simulink model "Quadcopter_State_model_Arduino"  (R2023b)
settings: Solver=VariableStepAuto  StartTime=0.0  StopTime=inf  FixedStep=0.00001  MinStep=0.001  RelTol=1e-3
model workspace (MAT data in the model file):
  DesiredPitchRoll : sugfis (value not decoded)
  DesiredThrust = sugfis
  DesiredThrust.Name = "fis"
  DesiredThrust.Type = "sugeno"
  DesiredThrust.AndMethod = "min"
  DesiredThrust.OrMethod = "max"
  DesiredThrust.FuzzyInferenceSystem.LocalImplicationMethod = "prod"
  DesiredThrust.FuzzyInferenceSystem.LocalAggregationMethod = "sum"
  DesiredThrust.FuzzyInferenceSystem.LocalDefuzzificationMethod = "wtaver"
  DesiredThrust.Inputs = fisvar
  DesiredThrust.Inputs.LocalName = "e_zdot"
  DesiredThrust.Inputs.Range = [-0.3 0.3]
  DesiredThrust.Inputs.EvalfisData.name = ' '
  DesiredThrust.Inputs.EvalfisData.range = [-0.3 0.3]
  DesiredThrust.Inputs.EvalfisData.mf(1).name = ' '
  DesiredThrust.Inputs.EvalfisData.mf(1).type = 'trimf'
  DesiredThrust.Inputs.EvalfisData.mf(1).params = [-0.45 -0.3 -0.15]
  DesiredThrust.Inputs.EvalfisData.mf(2).name = ' '
  DesiredThrust.Inputs.EvalfisData.mf(2).type = 'trimf'
  DesiredThrust.Inputs.EvalfisData.mf(2).params = [-0.3 -0.15 0]
  DesiredThrust.Inputs.EvalfisData.mf(3).name = ' '
  DesiredThrust.Inputs.EvalfisData.mf(3).type = 'trimf'
  DesiredThrust.Inputs.EvalfisData.mf(3).params = [-0.15 0 0.15]
  DesiredThrust.Inputs.EvalfisData.mf(4).name = ' '
  DesiredThrust.Inputs.EvalfisData.mf(4).type = 'trimf'
  DesiredThrust.Inputs.EvalfisData.mf(4).params = [0 0.15 0.3]
  DesiredThrust.Inputs.EvalfisData.mf(5).name = ' '
  DesiredThrust.Inputs.EvalfisData.mf(5).type = 'trimf'
  DesiredThrust.Inputs.EvalfisData.mf(5).params = [0.15 0.3 0.45]
  DesiredThrust.Inputs.LocalMembershipFunctions(1) = fismf
  DesiredThrust.Inputs.LocalMembershipFunctions(1).Function : function handle (value not decoded)
  DesiredThrust.Inputs.LocalMembershipFunctions(1).Parameters = [-0.45 -0.3 -0.15]
  DesiredThrust.Inputs.LocalMembershipFunctions(1).ParameterValueValidator : function handle (value not decoded)
  DesiredThrust.Inputs.LocalMembershipFunctions(1).NumParameters = 3
  DesiredThrust.Inputs.LocalMembershipFunctions(1).TypeStr = "trimf"
  DesiredThrust.Inputs.LocalMembershipFunctions(1).EvalfisData.name = ' '
  DesiredThrust.Inputs.LocalMembershipFunctions(1).EvalfisData.type = 'trimf'
  DesiredThrust.Inputs.LocalMembershipFunctions(1).EvalfisData.params = [-0.45 -0.3 -0.15]
  DesiredThrust.Inputs.LocalMembershipFunctions(1).fuzzy.internal.fis.MembershipFunction.LocalName = "StrongThrustDown"
  DesiredThrust.Inputs.LocalMembershipFunctions(1).UnmatchedInputArguments = struct()
  DesiredThrust.Inputs.LocalMembershipFunctions(2) = fismf
  DesiredThrust.Inputs.LocalMembershipFunctions(2).Function : function handle (value not decoded)
  DesiredThrust.Inputs.LocalMembershipFunctions(2).Parameters = [-0.3 -0.15 0]
  DesiredThrust.Inputs.LocalMembershipFunctions(2).ParameterValueValidator : function handle (value not decoded)
  DesiredThrust.Inputs.LocalMembershipFunctions(2).NumParameters = 3
  DesiredThrust.Inputs.LocalMembershipFunctions(2).TypeStr = "trimf"
  DesiredThrust.Inputs.LocalMembershipFunctions(2).EvalfisData.name = ' '
  DesiredThrust.Inputs.LocalMembershipFunctions(2).EvalfisData.type = 'trimf'
  DesiredThrust.Inputs.LocalMembershipFunctions(2).EvalfisData.params = [-0.3 -0.15 0]
  DesiredThrust.Inputs.LocalMembershipFunctions(2).fuzzy.internal.fis.MembershipFunction.LocalName = "MediumThrustDown"
  DesiredThrust.Inputs.LocalMembershipFunctions(2).UnmatchedInputArguments = struct()
  DesiredThrust.Inputs.LocalMembershipFunctions(3) = fismf
  DesiredThrust.Inputs.LocalMembershipFunctions(3).Function : function handle (value not decoded)
  DesiredThrust.Inputs.LocalMembershipFunctions(3).Parameters = [-0.15 0 0.15]
  DesiredThrust.Inputs.LocalMembershipFunctions(3).ParameterValueValidator : function handle (value not decoded)
  DesiredThrust.Inputs.LocalMembershipFunctions(3).NumParameters = 3
  DesiredThrust.Inputs.LocalMembershipFunctions(3).TypeStr = "trimf"
  DesiredThrust.Inputs.LocalMembershipFunctions(3).EvalfisData.name = ' '
  DesiredThrust.Inputs.LocalMembershipFunctions(3).EvalfisData.type = 'trimf'
  DesiredThrust.Inputs.LocalMembershipFunctions(3).EvalfisData.params = [-0.15 0 0.15]
  DesiredThrust.Inputs.LocalMembershipFunctions(3).fuzzy.internal.fis.MembershipFunction.LocalName = "NeutralThrust"
  DesiredThrust.Inputs.LocalMembershipFunctions(3).UnmatchedInputArguments = struct()
  DesiredThrust.Inputs.LocalMembershipFunctions(4) = fismf
  DesiredThrust.Inputs.LocalMembershipFunctions(4).Function : function handle (value not decoded)
  DesiredThrust.Inputs.LocalMembershipFunctions(4).Parameters = [0 0.15 0.3]
  DesiredThrust.Inputs.LocalMembershipFunctions(4).ParameterValueValidator : function handle (value not decoded)
  DesiredThrust.Inputs.LocalMembershipFunctions(4).NumParameters = 3
  DesiredThrust.Inputs.LocalMembershipFunctions(4).TypeStr = "trimf"
  DesiredThrust.Inputs.LocalMembershipFunctions(4).EvalfisData.name = ' '
  DesiredThrust.Inputs.LocalMembershipFunctions(4).EvalfisData.type = 'trimf'
  DesiredThrust.Inputs.LocalMembershipFunctions(4).EvalfisData.params = [0 0.15 0.3]
  DesiredThrust.Inputs.LocalMembershipFunctions(4).fuzzy.internal.fis.MembershipFunction.LocalName = "WeakThrustUp"
  DesiredThrust.Inputs.LocalMembershipFunctions(4).UnmatchedInputArguments = struct()
  DesiredThrust.Inputs.LocalMembershipFunctions(5) = fismf
  DesiredThrust.Inputs.LocalMembershipFunctions(5).Function : function handle (value not decoded)
  DesiredThrust.Inputs.LocalMembershipFunctions(5).Parameters = [0.15 0.3 0.45]
  DesiredThrust.Inputs.LocalMembershipFunctions(5).ParameterValueValidator : function handle (value not decoded)
  DesiredThrust.Inputs.LocalMembershipFunctions(5).NumParameters = 3
  DesiredThrust.Inputs.LocalMembershipFunctions(5).TypeStr = "trimf"
  DesiredThrust.Inputs.LocalMembershipFunctions(5).EvalfisData.name = ' '
  DesiredThrust.Inputs.LocalMembershipFunctions(5).EvalfisData.type = 'trimf'
  DesiredThrust.Inputs.LocalMembershipFunctions(5).EvalfisData.params = [0.15 0.3 0.45]
  DesiredThrust.Inputs.LocalMembershipFunctions(5).fuzzy.internal.fis.MembershipFunction.LocalName = "StrongThrustUp"
  DesiredThrust.Inputs.LocalMembershipFunctions(5).UnmatchedInputArguments = struct()
  DesiredThrust.Outputs = fisvar
  DesiredThrust.Outputs.LocalName = "DesiredThrust"
  DesiredThrust.Outputs.Range = [0 255]
  DesiredThrust.Outputs.EvalfisData.name = ' '
  DesiredThrust.Outputs.EvalfisData.range = [0 255]
  DesiredThrust.Outputs.EvalfisData.mf(1).name = ' '
  DesiredThrust.Outputs.EvalfisData.mf(1).type = 'constant'
  DesiredThrust.Outputs.EvalfisData.mf(1).params = 0
  DesiredThrust.Outputs.EvalfisData.mf(2).name = ' '
  DesiredThrust.Outputs.EvalfisData.mf(2).type = 'constant'
  DesiredThrust.Outputs.EvalfisData.mf(2).params = 63
  DesiredThrust.Outputs.EvalfisData.mf(3).name = ' '
  DesiredThrust.Outputs.EvalfisData.mf(3).type = 'constant'
  DesiredThrust.Outputs.EvalfisData.mf(3).params = 127
  DesiredThrust.Outputs.EvalfisData.mf(4).name = ' '
  DesiredThrust.Outputs.EvalfisData.mf(4).type = 'constant'
  DesiredThrust.Outputs.EvalfisData.mf(4).params = 191
  DesiredThrust.Outputs.EvalfisData.mf(5).name = ' '
  DesiredThrust.Outputs.EvalfisData.mf(5).type = 'constant'
  DesiredThrust.Outputs.EvalfisData.mf(5).params = 255
  DesiredThrust.Outputs.LocalMembershipFunctions(1) = fismf
  DesiredThrust.Outputs.LocalMembershipFunctions(1).Function : function handle (value not decoded)
  DesiredThrust.Outputs.LocalMembershipFunctions(1).Parameters = 0
  DesiredThrust.Outputs.LocalMembershipFunctions(1).ParameterValueValidator : function handle (value not decoded)
  DesiredThrust.Outputs.LocalMembershipFunctions(1).NumParameters = -1
  DesiredThrust.Outputs.LocalMembershipFunctions(1).TypeStr = "constant"
  DesiredThrust.Outputs.LocalMembershipFunctions(1).EvalfisData.name = ' '
  DesiredThrust.Outputs.LocalMembershipFunctions(1).EvalfisData.type = 'constant'
  DesiredThrust.Outputs.LocalMembershipFunctions(1).EvalfisData.params = 0
  DesiredThrust.Outputs.LocalMembershipFunctions(1).fuzzy.internal.fis.MembershipFunction.LocalName = "Weakest"
  DesiredThrust.Outputs.LocalMembershipFunctions(1).UnmatchedInputArguments = struct()
  DesiredThrust.Outputs.LocalMembershipFunctions(2) = fismf
  DesiredThrust.Outputs.LocalMembershipFunctions(2).Function : function handle (value not decoded)
  DesiredThrust.Outputs.LocalMembershipFunctions(2).Parameters = 63
  DesiredThrust.Outputs.LocalMembershipFunctions(2).ParameterValueValidator : function handle (value not decoded)
  DesiredThrust.Outputs.LocalMembershipFunctions(2).NumParameters = -1
  DesiredThrust.Outputs.LocalMembershipFunctions(2).TypeStr = "constant"
  DesiredThrust.Outputs.LocalMembershipFunctions(2).EvalfisData.name = ' '
  DesiredThrust.Outputs.LocalMembershipFunctions(2).EvalfisData.type = 'constant'
  DesiredThrust.Outputs.LocalMembershipFunctions(2).EvalfisData.params = 63
  DesiredThrust.Outputs.LocalMembershipFunctions(2).fuzzy.internal.fis.MembershipFunction.LocalName = "MediumWeak"
  DesiredThrust.Outputs.LocalMembershipFunctions(2).UnmatchedInputArguments = struct()
  DesiredThrust.Outputs.LocalMembershipFunctions(3) = fismf
  DesiredThrust.Outputs.LocalMembershipFunctions(3).Function : function handle (value not decoded)
  DesiredThrust.Outputs.LocalMembershipFunctions(3).Parameters = 127
  DesiredThrust.Outputs.LocalMembershipFunctions(3).ParameterValueValidator : function handle (value not decoded)
  DesiredThrust.Outputs.LocalMembershipFunctions(3).NumParameters = -1
  DesiredThrust.Outputs.LocalMembershipFunctions(3).TypeStr = "constant"
  DesiredThrust.Outputs.LocalMembershipFunctions(3).EvalfisData.name = ' '
  DesiredThrust.Outputs.LocalMembershipFunctions(3).EvalfisData.type = 'constant'
  DesiredThrust.Outputs.LocalMembershipFunctions(3).EvalfisData.params = 127
  DesiredThrust.Outputs.LocalMembershipFunctions(3).fuzzy.internal.fis.MembershipFunction.LocalName = "Nuetral"
  DesiredThrust.Outputs.LocalMembershipFunctions(3).UnmatchedInputArguments = struct()
  DesiredThrust.Outputs.LocalMembershipFunctions(4) = fismf
  DesiredThrust.Outputs.LocalMembershipFunctions(4).Function : function handle (value not decoded)
  DesiredThrust.Outputs.LocalMembershipFunctions(4).Parameters = 191
  DesiredThrust.Outputs.LocalMembershipFunctions(4).ParameterValueValidator : function handle (value not decoded)
  DesiredThrust.Outputs.LocalMembershipFunctions(4).NumParameters = -1
  DesiredThrust.Outputs.LocalMembershipFunctions(4).TypeStr = "constant"
  DesiredThrust.Outputs.LocalMembershipFunctions(4).EvalfisData.name = ' '
  DesiredThrust.Outputs.LocalMembershipFunctions(4).EvalfisData.type = 'constant'
  DesiredThrust.Outputs.LocalMembershipFunctions(4).EvalfisData.params = 191
  DesiredThrust.Outputs.LocalMembershipFunctions(4).fuzzy.internal.fis.MembershipFunction.LocalName = "MediumStrong"
  DesiredThrust.Outputs.LocalMembershipFunctions(4).UnmatchedInputArguments = struct()
  DesiredThrust.Outputs.LocalMembershipFunctions(5) = fismf
  DesiredThrust.Outputs.LocalMembershipFunctions(5).Function : function handle (value not decoded)
  DesiredThrust.Outputs.LocalMembershipFunctions(5).Parameters = 255
  DesiredThrust.Outputs.LocalMembershipFunctions(5).ParameterValueValidator : function handle (value not decoded)
  DesiredThrust.Outputs.LocalMembershipFunctions(5).NumParameters = -1
  DesiredThrust.Outputs.LocalMembershipFunctions(5).TypeStr = "constant"
  DesiredThrust.Outputs.LocalMembershipFunctions(5).EvalfisData.name = ' '
  DesiredThrust.Outputs.LocalMembershipFunctions(5).EvalfisData.type = 'constant'
  DesiredThrust.Outputs.LocalMembershipFunctions(5).EvalfisData.params = 255
  DesiredThrust.Outputs.LocalMembershipFunctions(5).fuzzy.internal.fis.MembershipFunction.LocalName = "Strongest"
  DesiredThrust.Outputs.LocalMembershipFunctions(5).UnmatchedInputArguments = struct()
  DesiredThrust.Rules(1) = fisrule
  DesiredThrust.Rules(1).LocalAntecedent = 1
  DesiredThrust.Rules(1).LocalConsequent = 5
  DesiredThrust.Rules(1).LocalDescription.input.name = "e_zdot"
  DesiredThrust.Rules(1).LocalDescription.input.mf = "StrongThrustDown"
  DesiredThrust.Rules(1).LocalDescription.input.complement = 0
  DesiredThrust.Rules(1).LocalDescription.output.name = "DesiredThrust"
  DesiredThrust.Rules(1).LocalDescription.output.mf = "Strongest"
  DesiredThrust.Rules(1).LocalDescription.output.complement = 0
  DesiredThrust.Rules(1).LocalDescription.weight = 1
  DesiredThrust.Rules(1).LocalDescription.connection = 1
  DesiredThrust.Rules(1).LocalWeight = 1
  DesiredThrust.Rules(1).LocalConnection = 1
  DesiredThrust.Rules(1).EvalfisData.antecedent = 1
  DesiredThrust.Rules(1).EvalfisData.consequent = 5
  DesiredThrust.Rules(1).EvalfisData.weight = 1
  DesiredThrust.Rules(1).EvalfisData.connection = 1
  DesiredThrust.Rules(2) = fisrule
  DesiredThrust.Rules(2).LocalAntecedent = 2
  DesiredThrust.Rules(2).LocalConsequent = 4
  DesiredThrust.Rules(2).LocalDescription.input.name = "e_zdot"
  DesiredThrust.Rules(2).LocalDescription.input.mf = "MediumThrustDown"
  DesiredThrust.Rules(2).LocalDescription.input.complement = 0
  DesiredThrust.Rules(2).LocalDescription.output.name = "DesiredThrust"
  DesiredThrust.Rules(2).LocalDescription.output.mf = "MediumStrong"
  DesiredThrust.Rules(2).LocalDescription.output.complement = 0
  DesiredThrust.Rules(2).LocalDescription.weight = 1
  DesiredThrust.Rules(2).LocalDescription.connection = 1
  DesiredThrust.Rules(2).LocalWeight = 1
  DesiredThrust.Rules(2).LocalConnection = 1
  DesiredThrust.Rules(2).EvalfisData.antecedent = 2
  DesiredThrust.Rules(2).EvalfisData.consequent = 4
  DesiredThrust.Rules(2).EvalfisData.weight = 1
  DesiredThrust.Rules(2).EvalfisData.connection = 1
  DesiredThrust.Rules(3) = fisrule
  DesiredThrust.Rules(3).LocalAntecedent = 3
  DesiredThrust.Rules(3).LocalConsequent = 3
  DesiredThrust.Rules(3).LocalDescription.input.name = "e_zdot"
  DesiredThrust.Rules(3).LocalDescription.input.mf = "NeutralThrust"
  DesiredThrust.Rules(3).LocalDescription.input.complement = 0
  DesiredThrust.Rules(3).LocalDescription.output.name = "DesiredThrust"
  DesiredThrust.Rules(3).LocalDescription.output.mf = "Nuetral"
  DesiredThrust.Rules(3).LocalDescription.output.complement = 0
  DesiredThrust.Rules(3).LocalDescription.weight = 1
  DesiredThrust.Rules(3).LocalDescription.connection = 1
  DesiredThrust.Rules(3).LocalWeight = 1
  DesiredThrust.Rules(3).LocalConnection = 1
  DesiredThrust.Rules(3).EvalfisData.antecedent = 3
  DesiredThrust.Rules(3).EvalfisData.consequent = 3
  DesiredThrust.Rules(3).EvalfisData.weight = 1
  DesiredThrust.Rules(3).EvalfisData.connection = 1
  DesiredThrust.Rules(4) = fisrule
  DesiredThrust.Rules(4).LocalAntecedent = 4
  DesiredThrust.Rules(4).LocalConsequent = 2
  DesiredThrust.Rules(4).LocalDescription.input.name = "e_zdot"
  DesiredThrust.Rules(4).LocalDescription.input.mf = "WeakThrustUp"
  DesiredThrust.Rules(4).LocalDescription.input.complement = 0
  DesiredThrust.Rules(4).LocalDescription.output.name = "DesiredThrust"
  DesiredThrust.Rules(4).LocalDescription.output.mf = "MediumWeak"
  DesiredThrust.Rules(4).LocalDescription.output.complement = 0
  DesiredThrust.Rules(4).LocalDescription.weight = 1
  DesiredThrust.Rules(4).LocalDescription.connection = 1
  DesiredThrust.Rules(4).LocalWeight = 1
  DesiredThrust.Rules(4).LocalConnection = 1
  DesiredThrust.Rules(4).EvalfisData.antecedent = 4
  DesiredThrust.Rules(4).EvalfisData.consequent = 2
  DesiredThrust.Rules(4).EvalfisData.weight = 1
  DesiredThrust.Rules(4).EvalfisData.connection = 1
  DesiredThrust.Rules(5) = fisrule
  DesiredThrust.Rules(5).LocalAntecedent = 5
  DesiredThrust.Rules(5).LocalConsequent = 1
  DesiredThrust.Rules(5).LocalDescription.input.name = "e_zdot"
  DesiredThrust.Rules(5).LocalDescription.input.mf = "StrongThrustUp"
  DesiredThrust.Rules(5).LocalDescription.input.complement = 0
  DesiredThrust.Rules(5).LocalDescription.output.name = "DesiredThrust"
  DesiredThrust.Rules(5).LocalDescription.output.mf = "Weakest"
  DesiredThrust.Rules(5).LocalDescription.output.complement = 0
  DesiredThrust.Rules(5).LocalDescription.weight = 1
  DesiredThrust.Rules(5).LocalDescription.connection = 1
  DesiredThrust.Rules(5).LocalWeight = 1
  DesiredThrust.Rules(5).LocalConnection = 1
  DesiredThrust.Rules(5).EvalfisData.antecedent = 5
  DesiredThrust.Rules(5).EvalfisData.consequent = 1
  DesiredThrust.Rules(5).EvalfisData.weight = 1
  DesiredThrust.Rules(5).EvalfisData.connection = 1
  DesiredThrust.EvalfisData.name = ' '
  DesiredThrust.EvalfisData.type = 'sugeno'
  DesiredThrust.EvalfisData.andMethod = 'min'
  DesiredThrust.EvalfisData.orMethod = 'max'
  DesiredThrust.EvalfisData.defuzzMethod = 'wtaver'
  DesiredThrust.EvalfisData.impMethod = 'prod'
  DesiredThrust.EvalfisData.aggMethod = 'sum'
  DesiredThrust.EvalfisData.input.name = ' '
  DesiredThrust.EvalfisData.input.range = [-0.3 0.3]
  DesiredThrust.EvalfisData.input.mf(1).name = ' '
  DesiredThrust.EvalfisData.input.mf(1).type = 'trimf'
  DesiredThrust.EvalfisData.input.mf(1).params = [-0.45 -0.3 -0.15]
  DesiredThrust.EvalfisData.input.mf(2).name = ' '
  DesiredThrust.EvalfisData.input.mf(2).type = 'trimf'
  DesiredThrust.EvalfisData.input.mf(2).params = [-0.3 -0.15 0]
  DesiredThrust.EvalfisData.input.mf(3).name = ' '
  DesiredThrust.EvalfisData.input.mf(3).type = 'trimf'
  DesiredThrust.EvalfisData.input.mf(3).params = [-0.15 0 0.15]
  DesiredThrust.EvalfisData.input.mf(4).name = ' '
  DesiredThrust.EvalfisData.input.mf(4).type = 'trimf'
  DesiredThrust.EvalfisData.input.mf(4).params = [0 0.15 0.3]
  DesiredThrust.EvalfisData.input.mf(5).name = ' '
  DesiredThrust.EvalfisData.input.mf(5).type = 'trimf'
  DesiredThrust.EvalfisData.input.mf(5).params = [0.15 0.3 0.45]
  DesiredThrust.EvalfisData.output.name = ' '
  DesiredThrust.EvalfisData.output.range = [0 255]
  DesiredThrust.EvalfisData.output.mf(1).name = ' '
  DesiredThrust.EvalfisData.output.mf(1).type = 'constant'
  DesiredThrust.EvalfisData.output.mf(1).params = 0
  DesiredThrust.EvalfisData.output.mf(2).name = ' '
  DesiredThrust.EvalfisData.output.mf(2).type = 'constant'
  DesiredThrust.EvalfisData.output.mf(2).params = 63
  DesiredThrust.EvalfisData.output.mf(3).name = ' '
  DesiredThrust.EvalfisData.output.mf(3).type = 'constant'
  DesiredThrust.EvalfisData.output.mf(3).params = 127
  DesiredThrust.EvalfisData.output.mf(4).name = ' '
  DesiredThrust.EvalfisData.output.mf(4).type = 'constant'
  DesiredThrust.EvalfisData.output.mf(4).params = 191
  DesiredThrust.EvalfisData.output.mf(5).name = ' '
  DesiredThrust.EvalfisData.output.mf(5).type = 'constant'
  DesiredThrust.EvalfisData.output.mf(5).params = 255
  DesiredThrust.EvalfisData.rule(1).antecedent = 1
  DesiredThrust.EvalfisData.rule(1).consequent = 5
  DesiredThrust.EvalfisData.rule(1).weight = 1
  DesiredThrust.EvalfisData.rule(1).connection = 1
  DesiredThrust.EvalfisData.rule(2).antecedent = 2
  DesiredThrust.EvalfisData.rule(2).consequent = 4
  DesiredThrust.EvalfisData.rule(2).weight = 1
  DesiredThrust.EvalfisData.rule(2).connection = 1
  DesiredThrust.EvalfisData.rule(3).antecedent = 3
  DesiredThrust.EvalfisData.rule(3).consequent = 3
  DesiredThrust.EvalfisData.rule(3).weight = 1
  DesiredThrust.EvalfisData.rule(3).connection = 1
  DesiredThrust.EvalfisData.rule(4).antecedent = 4
  DesiredThrust.EvalfisData.rule(4).consequent = 2
  DesiredThrust.EvalfisData.rule(4).weight = 1
  DesiredThrust.EvalfisData.rule(4).connection = 1
  DesiredThrust.EvalfisData.rule(5).antecedent = 5
  DesiredThrust.EvalfisData.rule(5).consequent = 1
  DesiredThrust.EvalfisData.rule(5).weight = 1
  DesiredThrust.EvalfisData.rule(5).connection = 1
  DesiredYaw : sugfis (value not decoded)
  Desired_Pitch = 0
  Desired_Roll = 0
  Desired_Yaw = 0
  Desired_Z_Velocity = -3
  FuzzyMotorspeed : sugfis (value not decoded)
values from neighbouring files (symbols this model uses):
  g = 9.81    [Quadcopter_Constants.m]
  Ixx = 0.0294838    [Quadcopter_Constants.m]
  Iyy = 0.0294838    [Quadcopter_Constants.m]
  Izz = 0.058967624    [Quadcopter_Constants.m]
  Jr = (6e-5)*1.358    (= 8.148e-05)    [Quadcopter_Constants.m]
  kd = 1    [Quadcopter_Constants.m]
  kd_phi = 1    [Quadcopter_Constants.m]
  kd_theta = 1    [Quadcopter_Constants.m]
  kf = 1    [Quadcopter_Constants.m]
  ki = 1    [Quadcopter_Constants.m]
  ki_phi = 1    [Quadcopter_Constants.m]
  ki_theta = 1    [Quadcopter_Constants.m]
  km = 4.74157e-9    (= 4.74157e-09)    [Quadcopter_Constants.m]
  kp = 1    [Quadcopter_Constants.m]
  kp_phi = 1    [Quadcopter_Constants.m]
  kp_theta = 1    [Quadcopter_Constants.m]
  kr = (0.1)*1.358    (= 0.1358)    [Quadcopter_Constants.m]
  kt = (0.1)*1.358    (= 0.1358)    [Quadcopter_Constants.m]
  l = 0.254    [Quadcopter_Constants.m]
  m = 0.914    [Quadcopter_Constants.m]
  sample_freq = 1000    [Quadcopter_Constants.m]
undefined symbols (not defined in the file or in its folder): LF
libraries: fuzblock x18, instrumentseriallib x12, simulink_extras x6, vrlib x4, instrumentlib x3, etargetslib x1, slpidlib x1, simulink x1
(part 1 of 5)
settings Model: ExtModeTrigDuration=2  Creator=benki  LastModifiedBy=User1
settings SolverCC: MaxConsecutiveMinStep=10
settings OptimizationCC: EnhancedBackFolding=on  PassReuseOutputArgsThreshold=0  MaxStackSize=64  OptimizeBlockOrder=speed  DifferentSizesBufferReuse=on  OptimizationCustomize=off
settings DebuggingCC: ParameterTunabilityLossMsg=error
settings HardwareCC: ProdBitPerInt=16  ProdBitPerPointer=16  ProdBitPerSizeT=16  ProdBitPerPtrDiffT=16  ProdLargestAtomicFloat=None  ProdWordSize=8  ProdHWDeviceType=Atmel->AVR  UseEmbeddedCoderFeatures=off  UseSimulinkCoderFeatures=off
settings ModelReferenceCC: EnableRefExpFcnMdlSchedulingChecks=on
settings SFSimCC: MATLABDynamicMemAlloc=off
settings RTWCC: Description=Embedded Coder  SystemTargetFile=ert.tlc  HardwareBoard=Arduino Mega 2560  TemplateMakefile=ert_default_tmf  Toolchain=Arduino AVR
settings CodeAppCC: ForceParamTrailComments=on  OperatorAnnotations=on
settings ERTTargetCC: ERTCustomFileBanners=off  SupportContinuousTime=on  SupportNonInlinedSFcns=on  RemoveResetFunc=off  SupportVariableSizeSignals=on  ModelStepFunctionPrototypeControlCompliant=off  ExtModeTransport=3  ExtModeStaticAlloc=on  ExtModeAutomaticAllocSize=off  ExtModeStaticAllocSize=2048  ExtModeMexFile=ext_xcp  ExtModeIntrfLevel=Level2 - Open

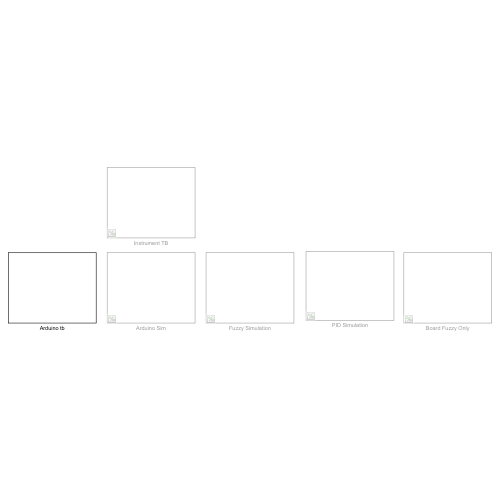
[thumbnail: Simulink's stored preview of the top-level diagram]
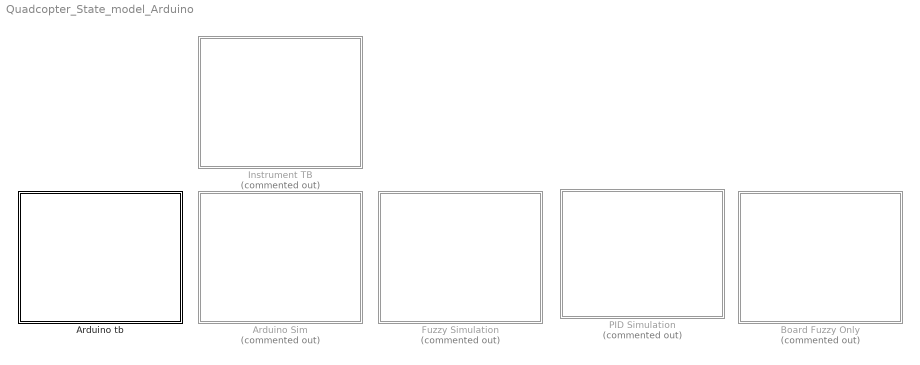
== system Quadcopter_State_model_Arduino ==
  Arduino Sim : Subsystem  Commented=on
  Arduino tb : Subsystem
  Board Fuzzy Only : Subsystem  Commented=on
  Fuzzy Simulation : Subsystem  Commented=on
  Instrument TB : Subsystem  Commented=on
  PID Simulation : Subsystem  Commented=on

== system Quadcopter_State_model_Arduino/Arduino Sim ==
  Arduino Communication : Subsystem
  Bus Selector : BusSelector  OutputSignals=phi,phi_dot,theta,theta_dot,psi,psi_dot,x,x_dot,y,y_dot,z,z_dot
  Control Panel : Subsystem
  Control Vector : Subsystem
  Gain{1..3,6} (4 alike) : Gain  Gain=4.372549019607  OutDataTypeStr=double
  Phi Scope : Scope
  Psi Scope : Scope
  Quadcopter Dynamics1 : Subsystem
  Relative Speed : Subsystem
  Scope : Scope  NumInputPorts=12
  Theta Scope : Scope
  Visualization : Subsystem  Commented=on
  Z Velocity Scope : Scope
  wires:
  Quadcopter Dynamics1/1(X_State) -> Visualization/1(X_State), Arduino Communication/1(X_State), Bus Selector/1
  Bus Selector/4 -> Scope/4  "<theta_dot>"
  Bus Selector/11 -> Scope/11  "<z>"
  Bus Selector/7 -> Scope/7  "<x>"
  Bus Selector/8 -> Scope/8  "<x_dot>"
  Bus Selector/10 -> Scope/10  "<y_dot>"
  Bus Selector/5 -> Psi Scope/1, Scope/5  "<psi>"
  Bus Selector/6 -> Scope/6  "<psi_dot>"
  Bus Selector/2 -> Scope/2  "<phi_dot>"
  Bus Selector/12 -> Z Velocity Scope/1, Scope/12  "<z_dot>"
  Bus Selector/1 -> Phi Scope/1, Scope/1  "<phi>"
  Bus Selector/3 -> Theta Scope/1, Scope/3  "<theta>"
  Bus Selector/9 -> Scope/9  "<y>"
  Relative Speed/1(Omega_R) -> Quadcopter Dynamics1/5(Omega_R)
  Control Vector/1(U1) -> Quadcopter Dynamics1/1(U1)
  Control Vector/2(U2) -> Quadcopter Dynamics1/2(U2)
  Control Vector/3(U3) -> Quadcopter Dynamics1/3(U3)
  Control Vector/4(U4) -> Quadcopter Dynamics1/4(U4)
  Gain1/1 -> Control Vector/1(Omega_1), Relative Speed/1(Omega_1)
  Gain2/1 -> Control Vector/2(Omega_2), Relative Speed/2(Omega_2)
  Gain3/1 -> Control Vector/3(Omega_3), Relative Speed/3(Omega_3)
  Gain6/1 -> Control Vector/4(Omega_4), Relative Speed/4(Omega_4)
  Arduino Communication/4(Omega_4) -> Gain6/1
  Arduino Communication/3(Omega_3) -> Gain3/1
  Arduino Communication/2(Omega_2) -> Gain2/1
  Arduino Communication/1(Omega_1) -> Gain1/1

== system Quadcopter_State_model_Arduino/Arduino tb ==
  Byte Pack : etargetslib/Byte Pack  datatypes={'single'}  byteAlign=4
  Cast To Single : DataTypeConversion  OutDataTypeStr=single  SaturateOnIntegerOverflow=off  RndMeth=Floor
  Constant : Constant  Value=[128 128 128 128 128 128 128 ]  OutDataTypeStr=single
  Display Data1 : Display
  Display Data2 : Display
  Serial Configuration : instrumentseriallib/Serial Configuration  Priority=-200000  PortSel=COM8  Port=COM8  ComPort=COM8  BaudRate=9600  DataBits=8  Parity=none  StopBits=1  ByteOrder=little-endian  FlowControl=none  Timeout=100  SimulateUsing=Interpreted execution  BlockInModel=on  aMode=1
  Serial Receive2 : instrumentseriallib/Serial Receive  Priority=1  PortSel=COM8  Port=COM8  ComPort=COM8  DataType=uint8  SaveDataType=uint8  ToggleHeader=off  Header=[]  ToggleTerminator=off  Terminator=LF ('\n')  CustomTerminator=[]  InputFormat=Column major  ToggleDataSize=on  DataSize=[1 5]  EnableBlockingMode=on  ActionDataUnavailable=Output last received value  ActionWhenDataUnavailable=Output last received value  CustomValue=0  SampleTime=0.01  SimulateUsing=Interpreted execution  BlockInModel=on  aMode=1
  Serial Send : instrumentseriallib/Serial Send  Priority=1  PortSel=COM8  Port=COM8  ComPort=COM8  Header=[]  Terminator=<none>  CustomTerminator=[]  EnableBlockingMode=on  SimulateUsing=Interpreted execution  BlockInModel=on  aMode=1
  Zero-Order Hold : ZeroOrderHold  SampleTime=.005
  wires:
  Constant/1 -> Zero-Order Hold/1
  Serial Receive2/1 -> Display Data1/1
  Byte Pack/1 -> Serial Send/1
  Cast To Single/1 -> Display Data2/1, Byte Pack/1
  Zero-Order Hold/1 -> Cast To Single/1

== system Quadcopter_State_model_Arduino/Board Fuzzy Only ==
  note: For some reason uncommenting this nukes performance in the Fuzzy sim
  Bus Selector : BusSelector  OutputSignals=phi,phi_dot,theta,theta_dot,psi,psi_dot,x,x_dot,y,y_dot,z,z_dot
  Control Vector : Subsystem
  Demux : Demux
  Fuzzy Control System : Subsystem  Commented=on
  Fuzzy Control System1 : Subsystem  Commented=on
  Fuzzy Control System2 : Subsystem
  Gain{1..4} (4 alike) : Gain  Gain=4.372549019607
  Phi Scope : Scope
  Psi Scope : Scope
  Quadcopter Dynamics1 : Subsystem
  Relative Speed : Subsystem
  Saturation{,1..3} (4 alike) : Saturate  UpperLimit=255  LowerLimit=0  OutMin=[0]  OutMax=[255]  OutDataTypeStr=uint8
  Saturation{4..7} (4 alike) : Saturate  UpperLimit=255  LowerLimit=0  OutMin=[0]  OutMax=[255]  OutDataTypeStr=double
  Scope : Scope  NumInputPorts=12
  Theta Scope : Scope
  Z Velocity Scope : Scope
  wires:
  Bus Selector/4 -> Scope/4  "<theta_dot>"
  Bus Selector/11 -> Scope/11  "<z>"
  Bus Selector/7 -> Scope/7  "<x>"
  Demux/2 -> Saturation1/1  "Omega2"
  Bus Selector/8 -> Scope/8  "<x_dot>"
  Bus Selector/10 -> Scope/10  "<y_dot>"
  Bus Selector/5 -> Psi Scope/1, Scope/5  "<psi>"
  Bus Selector/6 -> Scope/6  "<psi_dot>"
  Bus Selector/2 -> Scope/2  "<phi_dot>"
  Demux/1 -> Saturation/1  "Omega1"
  Bus Selector/12 -> Z Velocity Scope/1, Scope/12  "<z_dot>"
  Bus Selector/1 -> Phi Scope/1, Scope/1  "<phi>"
  Bus Selector/3 -> Theta Scope/1, Scope/3  "<theta>"
  Demux/4 -> Saturation3/1  "Omega4"
  Bus Selector/9 -> Scope/9  "<y>"
  Relative Speed/1(Omega_R) -> Quadcopter Dynamics1/5(Omega_R)
  Control Vector/1(U1) -> Quadcopter Dynamics1/1(U1)
  Control Vector/2(U2) -> Quadcopter Dynamics1/2(U2)
  Control Vector/3(U3) -> Quadcopter Dynamics1/3(U3)
  Control Vector/4(U4) -> Quadcopter Dynamics1/4(U4)
  Saturation/1 -> Saturation4/1
  Saturation3/1 -> Saturation7/1
  Saturation5/1 -> Gain2/1
  Saturation4/1 -> Gain1/1
  Saturation7/1 -> Gain4/1
  Saturation6/1 -> Gain3/1
  Gain1/1 -> Control Vector/1(Omega_1), Relative Speed/1(Omega_1)
  Gain2/1 -> Control Vector/2(Omega_2), Relative Speed/2(Omega_2)
  Gain3/1 -> Control Vector/3(Omega_3), Relative Speed/3(Omega_3)
  Gain4/1 -> Control Vector/4(Omega_4), Relative Speed/4(Omega_4)
  Saturation1/1 -> Saturation5/1
  Saturation2/1 -> Saturation6/1
  Demux/3 -> Saturation2/1  "Omega3"
  Fuzzy Control System2/1(motorspeeds) -> Demux/1
  Quadcopter Dynamics1/1(X_State) -> Fuzzy Control System2/1(x_state), Bus Selector/1

== system Quadcopter_State_model_Arduino/Fuzzy Simulation ==
  note: For some reason uncommenting this nukes performance in the Fuzzy sim
  Arduino Communication : Subsystem
  Bus Selector : BusSelector  OutputSignals=phi,phi_dot,theta,theta_dot,psi,psi_dot,x,x_dot,y,y_dot,z,z_dot
  Control Vector : Subsystem
  Demux : Demux
  Fuzzy Control System : Subsystem  Commented=on
  Fuzzy Control System1 : Subsystem  Commented=on
  Fuzzy Control System2 : Subsystem
  Gain{1..4} (4 alike) : Gain  Gain=4.372549019607
  Phi Scope : Scope
  Psi Scope : Scope
  Quadcopter Dynamics1 : Subsystem
  Relative Speed : Subsystem
  Saturation{,1..3} (4 alike) : Saturate  UpperLimit=255  LowerLimit=0  OutMin=[0]  OutMax=[255]  OutDataTypeStr=uint8
  Saturation{4..7} (4 alike) : Saturate  UpperLimit=255  LowerLimit=0  OutMin=[0]  OutMax=[255]  OutDataTypeStr=double
  Scope : Scope  NumInputPorts=12
  Sensors : Subsystem
  Theta Scope : Scope
  Z Velocity Scope : Scope
  wires:
  Quadcopter Dynamics1/1(X_State) -> Sensors/1(X_State), Bus Selector/1
  Bus Selector/4 -> Scope/4  "<theta_dot>"
  Bus Selector/11 -> Scope/11  "<z>"
  Bus Selector/7 -> Scope/7  "<x>"
  Demux/2 -> Saturation1/1  "Omega2"
  Bus Selector/8 -> Scope/8  "<x_dot>"
  Bus Selector/10 -> Scope/10  "<y_dot>"
  Bus Selector/5 -> Psi Scope/1, Scope/5  "<psi>"
  Bus Selector/6 -> Scope/6  "<psi_dot>"
  Bus Selector/2 -> Scope/2  "<phi_dot>"
  Demux/1 -> Saturation/1  "Omega1"
  Bus Selector/12 -> Z Velocity Scope/1, Scope/12  "<z_dot>"
  Bus Selector/1 -> Phi Scope/1, Scope/1  "<phi>"
  Bus Selector/3 -> Theta Scope/1, Scope/3  "<theta>"
  Demux/4 -> Saturation3/1  "Omega4"
  Bus Selector/9 -> Scope/9  "<y>"
  Relative Speed/1(Omega_R) -> Quadcopter Dynamics1/5(Omega_R)
  Control Vector/1(U1) -> Quadcopter Dynamics1/1(U1)
  Control Vector/2(U2) -> Quadcopter Dynamics1/2(U2)
  Control Vector/3(U3) -> Quadcopter Dynamics1/3(U3)
  Control Vector/4(U4) -> Quadcopter Dynamics1/4(U4)
  Saturation/1 -> Saturation4/1
  Saturation3/1 -> Saturation7/1
  Saturation5/1 -> Gain2/1
  Saturation4/1 -> Gain1/1
  Saturation7/1 -> Gain4/1
  Saturation6/1 -> Gain3/1
  Gain1/1 -> Control Vector/1(Omega_1), Relative Speed/1(Omega_1)
  Gain2/1 -> Control Vector/2(Omega_2), Relative Speed/2(Omega_2)
  Gain3/1 -> Control Vector/3(Omega_3), Relative Speed/3(Omega_3)
  Gain4/1 -> Control Vector/4(Omega_4), Relative Speed/4(Omega_4)
  Saturation1/1 -> Saturation5/1
  Saturation2/1 -> Saturation6/1
  Demux/3 -> Saturation2/1  "Omega3"
  Fuzzy Control System2/1(motorspeeds) -> Demux/1
  Sensors/1(X_State Sensor) -> Arduino Communication/1(X_State), Fuzzy Control System2/1(x_state)

== system Quadcopter_State_model_Arduino/Instrument TB ==
  Constant : Constant  Value=[128 128 128 128 128 128 128 ]  OutDataTypeStr=single
  Display Data1 : Display
  Display Data2 : Display
  Query Instrument : instrumentlib/Query Instrument  sampleTime=.01  isWorkspaceObject=on  timeout=10  inputBufferSize=512  protocol=Serial  serialPort=COM1  baudRate=9600  gpibVendor=Keysight Technologies  boardIndex=0  primaryAddress=1  secondaryAddress=0  visaVendor=Keysight  visaSerialPort=0  chassisIndex=0  logicalAddress=0  tcpRemoteHost='127.0.0.1'  tcpRemotePort=4500  udpRemoteHost='127.0.0.1'  udpRemotePort=9090  visaTCPBoardIndex=0  visaTCPRemoteHost='127.0.0.1'  usbBoardIndex=0  usbManufID=0  usbModelCode=0  usbSerialNumber=0  wsVariableName=device  initAction=None  initCommand='DATA:SOURCE CH1'  initFunction=get  queryCommand='curve?'  responseFormat=ASCII  asciiFormatting='%d,'  precision=8-bit integer  byteOrder=Little endian  valuesToRead=1  removeBytes=off  afterOutputAction=Repeat query for new data  enableFrames=off  frameSize=1
  To Instrument : instrumentlib/To Instrument  sampleTime=.01  isWorkspaceObject=on  timeout=10  inputBufferSize=8192  protocol=Serial  serialPort=COM1  baudRate=9600  gpibVendor=ICS Electronics  boardIndex=0  primaryAddress=1  secondaryAddress=0  visaVendor=Keysight  visaSerialPort=0  chassisIndex=0  logicalAddress=0  tcpRemoteHost='127.0.0.1'  tcpRemotePort=4500  udpRemoteHost='127.0.0.1'  udpRemotePort=9090  visaTCPBoardIndex=0  visaTCPRemoteHost='127.0.0.1'  usbBoardIndex=0  usbManufID=0  usbModelCode=0  usbSerialNumber=0  wsVariableName=device  initAction=None  initCommand='DATA:SOURCE CH1'  initFunction=get  command=''  sendFormat=ASCII  asciiFormatting='%d'  precision=8-bit integer  byteOrder=Little endian
  wires:
  Constant/1 -> To Instrument/1, Display Data2/1
  Query Instrument/1 -> Display Data1/1

== system Quadcopter_State_model_Arduino/PID Simulation ==
  Bus Selector : BusSelector  OutputSignals=phi,phi_dot,theta,theta_dot,psi,psi_dot,x,x_dot,y,y_dot,z,z_dot
  Control Panel : Subsystem
  Controller_Subsystem : Subsystem
  Motor_speed : Subsystem
  Quadcopter Dynamics : Subsystem
  Relative Speed : Subsystem
  Scope : Scope  NumInputPorts=12
  Sensors : Subsystem
  Visualization : Subsystem
  wires:
  Quadcopter Dynamics/1(X_State) -> Sensors/1(X_State), Visualization/1(X_State), Bus Selector/1
  Bus Selector/4 -> Scope/4  "<theta_dot>"
  Bus Selector/11 -> Scope/11  "<z>"
  Bus Selector/7 -> Scope/7  "<x>"
  Motor_speed/2(Omega_2) -> Relative Speed/2(Omega_2)
  Bus Selector/8 -> Scope/8  "<x_dot>"
  Bus Selector/10 -> Scope/10  "<y_dot>"
  Bus Selector/5 -> Scope/5  "<psi>"
  Bus Selector/6 -> Scope/6  "<psi_dot>"
  Bus Selector/2 -> Scope/2  "<phi_dot>"
  Controller_Subsystem/1(U1) -> Motor_speed/1(U1), Quadcopter Dynamics/1(U1)
  Motor_speed/1(Omega_1) -> Relative Speed/1(Omega_1)
  Controller_Subsystem/3(U3) -> Motor_speed/3(U3), Quadcopter Dynamics/3(U3)
  Bus Selector/12 -> Scope/12  "<z_dot>"
  Controller_Subsystem/2(U2) -> Motor_speed/2(U2), Quadcopter Dynamics/2(U2)
  Motor_speed/3(Omega_3) -> Relative Speed/3(Omega_3)
  Controller_Subsystem/4(U4) -> Motor_speed/4(U4), Quadcopter Dynamics/4(U4)
  Bus Selector/1 -> Scope/1  "<phi>"
  Bus Selector/3 -> Scope/3  "<theta>"
  Motor_speed/4(Omega_4) -> Relative Speed/4(Omega_4)
  Bus Selector/9 -> Scope/9  "<y>"
  Relative Speed/1(Omega_R) -> Quadcopter Dynamics/5(Omega_R)
  Sensors/1(X_State Sensor) -> Controller_Subsystem/1(X_State)

== system Quadcopter_State_model_Arduino/Arduino Sim/Arduino Communication ==
  X_State : Inport
  Bus Selector : BusSelector  OutputSignals=theta,phi,psi,z_dot,theta_dot,phi_dot,psi_dot
  Cast To Single{,1..6} (7 alike) : DataTypeConversion  OutDataTypeStr=single  SaturateOnIntegerOverflow=off  RndMeth=Floor
  Desired Pitch : Constant  Value=0  OutDataTypeStr=single
  Desired Roll : Constant  Value=0  OutDataTypeStr=single
  Desired Yaw : Constant  Value=0  OutDataTypeStr=single
  Desired Z Velocity : Constant  Value=0  OutDataTypeStr=single
  Display : Display
  Display1 : Display
  Gain : Gain  Gain=pi  OutDataTypeStr=single
  Gain1 : Gain  Gain=pi  OutDataTypeStr=single
  Gain2 : Gain  Gain=pi  OutDataTypeStr=single
  MATLAB Function : MATLAB Function  TreatAsAtomicUnit=on
  Matrix Concatenate : Concatenate  NumInputs=11  ConcatenateDimension=2
  Radians to Degrees : simulink_extras/Transformations/Radians to Degrees
  Radians to Degrees1 : simulink_extras/Transformations/Radians to Degrees
  Radians to Degrees2 : simulink_extras/Transformations/Radians to Degrees
  Serial Configuration : instrumentseriallib/Serial Configuration  Priority=-200000  PortSel=COM15  Port=COM15  ComPort=COM15  BaudRate=9600  DataBits=8  Parity=none  StopBits=1  ByteOrder=little-endian  FlowControl=none  Timeout=10  SimulateUsing=Interpreted execution  BlockInModel=on  aMode=1
  Serial Receive : instrumentseriallib/Serial Receive  Priority=1  PortSel=COM15  Port=COM15  ComPort=COM15  DataType=uint8  SaveDataType=uint8  ToggleHeader=off  Header=[]  ToggleTerminator=off  Terminator=<none>  CustomTerminator=[]  InputFormat=Column major  ToggleDataSize=on  DataSize=[1 4]  EnableBlockingMode=on  ActionDataUnavailable=Output last received value  ActionWhenDataUnavailable=Output last received value  CustomValue=0  SampleTime=0.01  SimulateUsing=Interpreted execution  BlockInModel=on  aMode=1
  Serial Send : instrumentseriallib/Serial Send  Priority=1  PortSel=COM15  Port=COM15  ComPort=COM15  Header=[]  Terminator=<none>  CustomTerminator=[]  EnableBlockingMode=on  SimulateUsing=Interpreted execution  BlockInModel=on  aMode=1
  Sin : Trigonometry
  Sin1 : Trigonometry
  Sin2 : Trigonometry
  Omega_1 : Outport
  Omega_2 : Outport  Port=2
  Omega_3 : Outport  Port=3
  Omega_4 : Outport  Port=4
  wires:
  X_State/1 -> Bus Selector/1
  Bus Selector/2 -> Cast To Single5/1  "<phi>"
  Bus Selector/4 -> Cast To Single/1  "<z_dot>"
  Bus Selector/3 -> Cast To Single6/1  "<psi>"
  Radians to Degrees/1 -> Matrix Concatenate/1  "roll_meas"
  Radians to Degrees1/1 -> Matrix Concatenate/2  "pitch_meas"
  Radians to Degrees2/1 -> Matrix Concatenate/3  "yaw_meas"
  Bus Selector/5 -> Cast To Single1/1  "<theta_dot>"
  Bus Selector/6 -> Cast To Single2/1  "<phi_dot>"
  Bus Selector/7 -> Cast To Single3/1  "<psi_dot>"
  Bus Selector/1 -> Cast To Single4/1  "<theta>"
  Sin/1 -> Gain/1
  Gain/1 -> Radians to Degrees/1
  Gain1/1 -> Radians to Degrees1/1
  Sin1/1 -> Gain1/1
  Gain2/1 -> Radians to Degrees2/1
  Sin2/1 -> Gain2/1
  MATLAB Function/1(m1o) -> Omega_1/1
  MATLAB Function/2(m2o) -> Omega_2/1
  MATLAB Function/3(m3o) -> Omega_3/1
  MATLAB Function/4(m4o) -> Omega_4/1
  Desired Yaw/1 -> Matrix Concatenate/10  "inputYaw"
  Desired Z Velocity/1 -> Matrix Concatenate/11  "inputZdot"
  Desired Pitch/1 -> Matrix Concatenate/9  "inputPitch"
  Desired Roll/1 -> Matrix Concatenate/8  "inputRoll"
  Matrix Concatenate/1 -> Display1/1, Serial Send/1
  Serial Receive/1 -> Display/1, MATLAB Function/1(m)
  Cast To Single/1 -> Matrix Concatenate/4
  Cast To Single1/1 -> Matrix Concatenate/5
  Cast To Single2/1 -> Matrix Concatenate/6
  Cast To Single3/1 -> Matrix Concatenate/7
  Cast To Single4/1 -> Sin/1
  Cast To Single5/1 -> Sin1/1
  Cast To Single6/1 -> Sin2/1
